simulink model "MRStandardSimulation"  (R2021a)
settings: Solver=VariableStepAuto  StartTime=0.0  StopTime=Tend  RelTol=1e-3
values from neighbouring files (symbols this model uses):
  F = 10    [MRStandardPlantLPMExample.m]
  J = [0 0 1;1 0 0;-1 1 0]    [MRStandardPlantLPMExample.m]
  K = 2    [MRStandardPlantLPMExample.m]    (also in SIMOLPMTest.m = [0.01*(1/(0.3*2*pi)*s+1)/(1/(3*2*pi)*s+1) 0.5 2/3])
  Pd = c2d(P,TsH)    [MRStandardPlantLPMExample.m]    (also in SIMOLPMTest.m = c2d(P,Ts,'zoh'))
  rH = [repmat(rH(1:end-1),per,1);rH(end)]    [MRStandardPlantLPMExample.m]    (also in MultiRateLPM.m = repmat(rp,Per,1); MultiratePFG.m = ra(:,k))
  TsH = 1/144    (= 0.00694444444444)    [MRStandardPlantLPMExample.m]    (also in MultiRateLPM.m = 0.005; MultiratePFG.m = 0.0025; unliftfrd.m = TsL/F; unliftfrdWithoutRep.m = GliftSIMO.Ts)
libraries: dspsrcs4 x1
settings Model: Creator=s152009  LastModifiedBy=s152009
settings DebuggingCC: AlgebraicLoopMsg=none

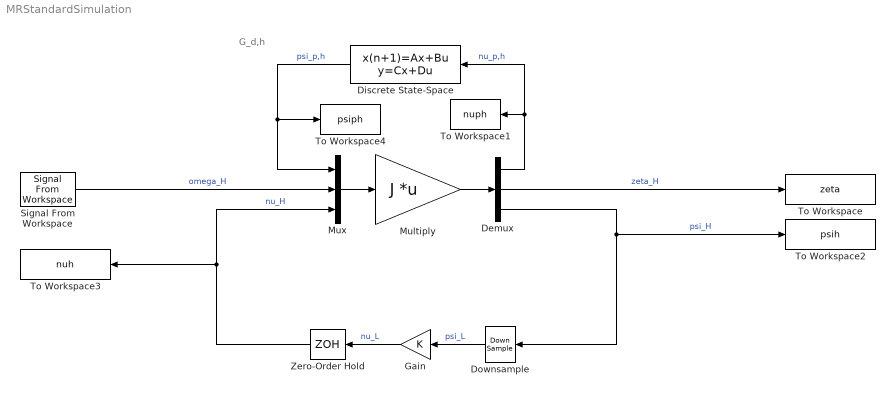
== system MRStandardSimulation ==
  note: G_d,h
  Demux : Demux  Outputs=3
  Discrete State-Space : DiscreteStateSpace  A=ss(Pd).A  B=ss(Pd).B  C=ss(Pd).C  D=ss(Pd).D  SampleTime=TsH
  Downsample : DownSample  N=F  RateOptions=Allow multirate processing
  Gain : Gain  Gain=K
  Multiply : Gain  Gain=J  Multiplication=Matrix(K*u) (u vector)
  Mux : Mux  Inputs=3
  Signal From Workspace : dspsrcs4/Signal From Workspace  X=real(rH)  Ts=TsH  nsamps=1  OutputAfterFinalValue=Setting to zero  ignoreOrWarnInputAndFrameLengths=off  OutputFrames=off
  To Workspace : ToWorkspace  VariableName=zeta  SampleTime=TsH
      settings: Save2DSignal=2-D array (concatenate along first dimension)
  To Workspace1 : ToWorkspace  VariableName=nuph  SampleTime=TsH
      settings: Save2DSignal=2-D array (concatenate along first dimension)
  To Workspace2 : ToWorkspace  VariableName=psih  SampleTime=TsH
      settings: Save2DSignal=2-D array (concatenate along first dimension)
  To Workspace3 : ToWorkspace  VariableName=nuh  SampleTime=TsH
      settings: Save2DSignal=2-D array (concatenate along first dimension)
  To Workspace4 : ToWorkspace  VariableName=psiph  SampleTime=TsH
      settings: Save2DSignal=2-D array (concatenate along first dimension)
  Zero-Order Hold : ZeroOrderHold  SampleTime=TsH
  wires:
  Mux/1 -> Multiply/1
  Multiply/1 -> Demux/1
  Demux/1 -> Discrete State-Space/1, To Workspace1/1  "nu_p,h"
  Discrete State-Space/1 -> Mux/1, To Workspace4/1  "psi_p,h"
  Zero-Order Hold/1 -> Mux/3, To Workspace3/1  "nu_H"
  Demux/3 -> To Workspace2/1, Downsample/1  "psi_H"
  Downsample/1 -> Gain/1  "psi_L"
  Gain/1 -> Zero-Order Hold/1  "nu_L"
  Signal From Workspace/1 -> Mux/2  "omega_H"
  Demux/2 -> To Workspace/1  "zeta_H"
